simulink model "partage_activitee_situee"  (Simulink 7.5)
settings: Solver=ode45  StartTime=0.0  StopTime=inf  RelTol=1e-3
settings Model: Creator=paris  LastModifiedBy=paris

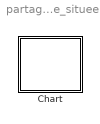
== system partage_activitee_situee ==
  Chart : Stateflow chart  TreatAsAtomicUnit=on

== stateflow chart Chart ==
  state MODEL_ACTIVITE_SITUEE
    state franchissement_VAG
      state Entree_Virage
      state Sortie_Virage
      state Approche_Virage
      state Fin_Gestion_Courbe
      state Debut_Gestion_Courbe
      MODEL_ACTIVITE_SITUEE.franchissement_VAG.Approche_Virage -> MODEL_ACTIVITE_SITUEE.franchissement_VAG.Entree_Virage : [ml.distPtA<=10]
      (default) -> MODEL_ACTIVITE_SITUEE.franchissement_VAG.Approche_Virage : [ml.distPtA<=50]
      MODEL_ACTIVITE_SITUEE.franchissement_VAG.Entree_Virage -> MODEL_ACTIVITE_SITUEE.franchissement_VAG.Debut_Gestion_Courbe : [ml.distPtA==0]
      MODEL_ACTIVITE_SITUEE.franchissement_VAG.Fin_Gestion_Courbe -> MODEL_ACTIVITE_SITUEE.franchissement_VAG.Sortie_Virage : [ml.distPtC==0]
      MODEL_ACTIVITE_SITUEE.franchissement_VAG.Debut_Gestion_Courbe -> MODEL_ACTIVITE_SITUEE.franchissement_VAG.Fin_Gestion_Courbe : [ml.distPtB==0]
    state Debut_Situation/
    state Fin_Situation
    state Gestion_obstacle
      state Evitemment
        state Fin_Evitement
        state Debut_Evitement
        Debut_Evitement -> Fin_Evitement : [ml.etat_obstacle==0]
        (default) -> Debut_Evitement : [ml.progression_SV==1]
      state Depassement
        state Fin_Depassement
        state Debut_Depassement
        state Suivi
        state Imminent
        Debut_Depassement -> Fin_Depassement : [ml.etat_obstacle==0]
        (default) -> Suivi
        Imminent -> Debut_Depassement : [ml.progression_SV==1]
        Suivi -> Imminent [order 1] : [ml.cligno==-1]
        Suivi -> Debut_Depassement [order 2] : [ml.progression_SV==1]
      state Approche_Obstacle
      Approche_Obstacle -> Evitemment [order 2] : [ml.sensCirculation_obstacle<>21]
      (default) -> Approche_Obstacle
      Approche_Obstacle -> Depassement [order 1] : [ml.sensCirculation_obstacle==21]
    state franchissement_VAD
      state Debut_Gestion_Courbe
      state Fin_Gestion_Courbe
      state Entree_Virage
      state Sortie_Virage
      state Approche_Virage
      MODEL_ACTIVITE_SITUEE.franchissement_VAD.Debut_Gestion_Courbe -> MODEL_ACTIVITE_SITUEE.franchissement_VAD.Fin_Gestion_Courbe : [ml.distPtB==0]
      MODEL_ACTIVITE_SITUEE.franchissement_VAD.Entree_Virage -> MODEL_ACTIVITE_SITUEE.franchissement_VAD.Debut_Gestion_Courbe : [ml.distPtA==0]
      MODEL_ACTIVITE_SITUEE.franchissement_VAD.Fin_Gestion_Courbe -> MODEL_ACTIVITE_SITUEE.franchissement_VAD.Sortie_Virage : [ml.distPtC==0]
      MODEL_ACTIVITE_SITUEE.franchissement_VAD.Approche_Virage -> MODEL_ACTIVITE_SITUEE.franchissement_VAD.Entree_Virage : [ml.distPtA<=10]
      (default) -> MODEL_ACTIVITE_SITUEE.franchissement_VAD.Approche_Virage : [ml.distPtA<=50]
    Debut_Situation -> franchissement_VAG [order 2] : [ml.type_infrastructure==60 || ml.type_infrastructure==61]
    MODEL_ACTIVITE_SITUEE.franchissement_VAG.Sortie_Virage -> Fin_Situation : [ml.type_infrastructure==62]
    Debut_Situation -> franchissement_VAD [order 3] : [ml.type_infrastructure==63 || ml.type_infrastructure==64]
    Debut_Situation -> Gestion_obstacle [order 1] : [ml.etat_obstacle>0]
    MODEL_ACTIVITE_SITUEE.franchissement_VAD.Sortie_Virage -> Fin_Situation : [ml.type_infrastructure==62]
    Fin_Depassement -> Fin_Situation : [ml.etat_SV==0]
    (default) -> Debut_Situation
    Fin_Evitement -> Fin_Situation : [ml.etat_SV==0]
